simulink model "MCity_cs_withAEBSBlock"  (R2017a)
settings: Solver=ode5  StartTime=0.0  StopTime=3.95  FixedStep=1/200  RelTol=1e-3
PreLoadFcn:
  | check_NUTS_defined;
  | 
  | assignin('base',['model_closed_' bdroot],false);
InitFcn:
  | PreScanExperimentInitFcn(bdroot)
StopFcn:
  | PreScanExperimentStopFcn(bdroot)
model workspace (MAT data in the model file):
  mbox_table : struct (value not decoded)
  model_closed = 0
  sim_status = 0
values from neighbouring files (symbols this model uses):
  d_offset = -18.15    [monocityTestLeftTurn.mat]    (also in simulation_leftTurn_PreScan.m = dl/vl*vh - 43 + R)
undefined symbols (not defined in the file or in its folder): DiscIntNeverNeededParam, warningInitialVelocity, x0
libraries: simulink x78, PreScanSimulinkLibrary x14, simulink_extras x10, PreScanUsefulBlocks x4
(part 1 of 12)
CloseFcn:
  | evalin('base',['clear model_closed_' bdroot]);
settings Model: Creator=PRESCAN  LastModifiedBy=zhaoding
settings DataIOCC: LimitDataPoints=on  SaveFormat=Array
settings OptimizationCC: ExpressionDepthLimit=2147483647  InitFltsAndDblsToZero=on  LifeSpan=inf
settings DebuggingCC: SaveWithParameterizedLinksMsg=none  UnderspecifiedInitializationDetection=Classic  MergeDetectMultiDrivingBlocksExec=none  SignalResolutionControl=TryResolveAllWithWarning  MultiTaskDSMMsg=warning  MultiTaskCondExecSysMsg=none  FcnCallInpInsideContextMsg=warning  StateNameClashWarn=warning  SFUnexpectedBacktrackingDiag=warning  SFNoUnconditionalDefaultTransitionDiag=warning  SFExecutionAtInitializationDiag=none
settings HardwareCC: ProdBitPerPointer=32  ProdBitPerSizeT=32  ProdBitPerPtrDiffT=32  ProdLargestAtomicFloat=None  ProdIntDivRoundTo=Undefined  ProdEndianess=Unspecified  ProdWordSize=32  ProdHWDeviceType=32-bit Generic
settings ModelReferenceCC: PropagateSignalLabelsOutOfModel=off
settings GRTTargetCC: TargetFcnLib=ansi_tfl_tmw.mat  TargetLangStandard=C89/C90 (ANSI)  GeneratePreprocessorConditionals=Disable all  CombineOutputUpdateFcns=off  GRTInterface=on
settings ConfigComp: CovMetricSettings=dw  CovHtmlReporting=on  CovSaveCumulativeToWorkspaceVar=on  CovSaveSingleToWorkspaceVar=on  CovExternalEMLEnable=off

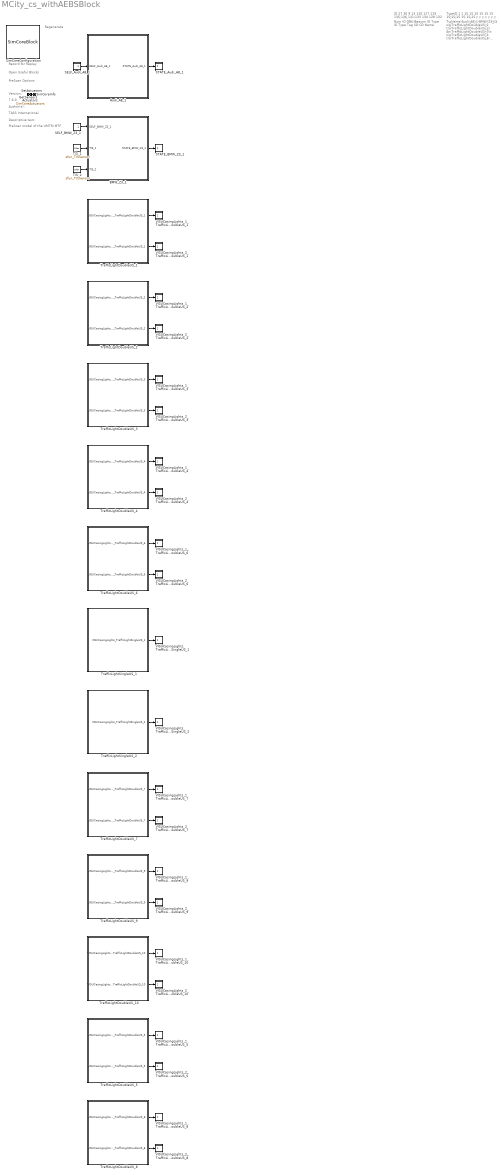
== system MCity_cs_withAEBSBlock ==
  note: Regenerate
  note: Record for Replay
  note: Open Useful Blocks
  note: PreScan Options
  note: Version:
  note: 7.6.0
  note: Author(s):
  note: TASS International
  note: Descriptive text:
  note: PreScan model of the UMTRI MTF.
  note: OBU-Beacon ID
  note: SD
      |
      | Y
      | Y
      | Y
      | Y
      | Y
      | Y
      | Y
      | Y
      | Y
      | Y
      | Y
      | Y
      | Y
      | Y
  note: CD
      |
      | N
      | N
      | N
      | N
      | N
      | N
      | N
      | N
      | N
      | N
      | N
      | N
      | N
      | N
  note: Num ID OBU-Beacon ID Type ID Type Tag SD CD Name
  note: TypeID
      |
      | 1
      | 1
      | 15
      | 15
      | 15
      | 15
      | 15
      | 15
      | 15
      | 15
      | 15
      | 15
      | 15
      | 15
  note: TypeTag
      |
      | Car
      | Car
      | Anim traffic sign
      | Anim traffic sign
      | Anim traffic sign
      | Anim traffic sign
      | Anim traffic sign
      | Anim traffic sign
      | Anim traffic sign
      | Anim traffic sign
      | Anim traffic sign
      | Anim traffic sign
      | Anim traffic sign
      | Anim traffic sign
  note: ID
      |
      | 27
      | 36
      | 9
      | 13
      | 126
      | 127
      | 129
      | 135
      | 136
      | 131
      | 133
      | 134
      | 128
      | 132
  note: Name
      |
      | Audi_A8_1
      | BMW_Z3_1
      | TrafficLightDoubleUS_1
      | TrafficLightDoubleUS_2
      | TrafficLightDoubleUS_3
      | TrafficLightDoubleUS_4
      | TrafficLightDoubleUS_6
      | TrafficLightSingleUS_1
      | TrafficLightSingleUS_2
      | TrafficLightDoubleUS_7
      | TrafficLightDoubleUS_9
      | TrafficLightDoubleUS_10
      | TrafficLightDoubleUS_5
      | TrafficLightDoubleUS_8
  Actuators : DataStoreMemory  Tag=Actuators  DataStoreName=SimCoreActuators  InitialValue=zeros(1086,1)  ShowAdditionalParam=off
      settings: DeleteFcn=PreScanBlockDeleteFcn;
  Audi_A8_1 : Subsystem  Tag=WorldObjectSubSystem  InitFcn=UniqueId = '11817';
      mask Display: image(imread('Audi_A8.jpg'));color('white');text(0,0,' ID=27\n')
  BMW_Z3_1 : Subsystem  Tag=WorldObjectSubSystem  InitFcn=|
      | UniqueId = '12190';
      | UniqueId = '12335';
      mask Display: image(imread('BMW_Z3.jpg'));color('white');text(0,0,' ID=36\n')
  GetSensors : Subsystem  Tag=GetSensors  Priority=2  mask(PreScan Simulation Core Block){NrOfSensors=16, TimeStep=1/200}
      mask prompts: NrOfSensors "Number of sensor values"; TimeStep "Timestep [s]"
      mask help:
      | Please do not remove this block from the PreScan compilation sheet,
      | as it contains essential configuration parameters for a PreScan simulation.
      settings: DeleteFcn=PreScanBlockDeleteFcn;
  SELF_Audi_A8_1 : Subsystem  Tag=SELF  Priority=3  mask(PreScan Source Block: SELF){PortName=SELF_Audi_A8_1, PortIndex=0, PortWidth=8, TimeStep=1/200}
      mask prompts: PortName "Auto-Assigned: Port Name [-]"; PortIndex "Auto-Assigned: Port Index [-]"; PortWidth "Auto-Assigned: Port Dimensions"; TimeStep "Auto-Assigned: Upload Period [s]"
      mask help:
      | The SELF port shows (state) information of the actor itself. The outputs are position in the experiment's axis system and the GPS coordinates, and the object's absolute velocity and compass heading.
      |
      | For more information, please click Help.
      settings: DeleteFcn=PreScanBlockDeleteFcn;
      mask Help: eval('openHelp(462)')
      mask Display: image(imread('GPS.png'))
  SELF_BMW_Z3_1 : Subsystem  Tag=SELF  Priority=3  mask(PreScan Source Block: SELF){PortName=SELF_BMW_Z3_1, PortIndex=8, PortWidth=8, TimeStep=1/200}
      mask prompts: PortName "Auto-Assigned: Port Name [-]"; PortIndex "Auto-Assigned: Port Index [-]"; PortWidth "Auto-Assigned: Port Dimensions"; TimeStep "Auto-Assigned: Upload Period [s]"
      mask help:
      | The SELF port shows (state) information of the actor itself. The outputs are position in the experiment's axis system and the GPS coordinates, and the object's absolute velocity and compass heading.
      |
      | For more information, please click Help.
      settings: DeleteFcn=PreScanBlockDeleteFcn;
      mask Help: eval('openHelp(462)')
      mask Display: image(imread('GPS.png'))
  STATE_Audi_A8_1 : Subsystem  Tag=State  Priority=0  mask(PreScan Sink Block: State){x0=-87.178748857646355, y0=373.9608626085182, z0=0.55, Roll0=0, Pitch0=0, Yaw0=92.476977617278507, TimeStep=1/200}
      mask prompts: x0 "Ini x-position VEHICLE wrt GLOBAL axis system [m]"; y0 "Ini y-position VEHICLE wrt GLOBAL axis system [m]"; z0 "Ini z-position VEHICLE wrt GLOBAL axis system [m]"; Roll0 "Ini roll-angle BODY wrt VEHICLE axis system [deg]"; Pitch0 "Ini pitch-angle BODY wrt VEHICLE axis system [deg]"; Yaw0 "Ini yaw-angle VEHICLE wrt GLOBAL axis system [deg]"; TimeStep "Time Step [s]"
      mask help:
      | The Actor State contains a vector signal of size (9x1), containing the following signals:
      |
      | -  Position                  (x,y,z)                                     [m]
      | -  Velocity                  (vx,vy,vz)                               [m/s]
      | -  Angles                    (Roll, Pitch, Yaw)                   [rad]
      |
      | The Actor state is defined in the global axis system.
      | The state is superponed on the Initial position defined in the GUI.
      |
      | For more information, please click Help.
      settings: DeleteFcn=PreScanBlockDeleteFcn;
      mask Help: eval('openHelp(222)')
      mask Display: image(imread('State.png'))
  STATE_BMW_Z3_1 : Subsystem  Tag=State  Priority=0  mask(PreScan Sink Block: State){x0=-92.980654036561049, y0=432.99562062308286, z0=0.4784, Roll0=0, Pitch0=0, Yaw0=271.20288231302447, TimeStep=1/200}
      mask prompts: x0 "Ini x-position VEHICLE wrt GLOBAL axis system [m]"; y0 "Ini y-position VEHICLE wrt GLOBAL axis system [m]"; z0 "Ini z-position VEHICLE wrt GLOBAL axis system [m]"; Roll0 "Ini roll-angle BODY wrt VEHICLE axis system [deg]"; Pitch0 "Ini pitch-angle BODY wrt VEHICLE axis system [deg]"; Yaw0 "Ini yaw-angle VEHICLE wrt GLOBAL axis system [deg]"; TimeStep "Time Step [s]"
      mask help:
      | The Actor State contains a vector signal of size (9x1), containing the following signals:
      |
      | -  Position                  (x,y,z)                                     [m]
      | -  Velocity                  (vx,vy,vz)                               [m/s]
      | -  Angles                    (Roll, Pitch, Yaw)                   [rad]
      |
      | The Actor state is defined in the global axis system.
      | The state is superponed on the Initial position defined in the GUI.
      |
      | For more information, please click Help.
      settings: DeleteFcn=PreScanBlockDeleteFcn;
      mask Help: eval('openHelp(222)')
      mask Display: image(imread('State.png'))
  SetActuators : Subsystem  Tag=SetActuators  Priority=1  mask(PreScan Simulation Core Block){TimeStep=1/200, NrOfActuators=1086}
      mask prompts: TimeStep "Timestep [s]"; NrOfActuators "Number of actuator values"
      mask help:
      | Please do not remove this block from the PreScan compilation sheet,
      | as it contains essential configuration parameters for a PreScan simulation.
      settings: DeleteFcn=PreScanBlockDeleteFcn;
  SimCoreConfiguration : M-S-Function  Tag=SimCoreConfiguration  Description=6A63ADE35867DA85095F0771801E5CBC5CA8CDFACC45876E9CB8251708310E18  FunctionName=SimCoreBlock  Parameters=ExperimentXML PortsXML SimulationCore HostName CheckStart EnableLog RfR EnableGPUAccel ShowComputationTime  mask(PreScan Simulation Core Configurator){SimulationCore=NUTS, HostName=0, CheckStart=0, prescanversion='7.6.0', EnableLog=off, RfR=0, EnableGPUAccel=off, ShowComputationTime=off}
      mask prompts: SimulationCore "Simulation Core"; HostName "Simulation Host"; CheckStart "Show START Dialog"; prescanversion "PreScan Version"; EnableLog "Create TA Log"; RfR "Record for Replay"; EnableGPUAccel "Enable GPU Acceleration"; ShowComputationTime "Show ComputationTime Scope"
      mask help:
      | Please do not remove this block from the PreScan compilation sheet,
      | as it contains essential configuration parameter for a PreScan simulation.
      mask init:
      | model = bdroot;
      | ExperimentXML = [model(1:end-3) '.pex'];
      | PortsXML = [model '_ports.pcd'];
      settings: DeleteFcn=PreScanBlockDeleteFcn;  ModelCloseFcn=assignin('base',['model_closed_' bdroot],true);
      mask Help: eval('openHelp(812)')
      mask Display: image(imread('prescanlogo.ico'))
  SimCoreInfo : Subsystem  Tag=SimCoreInfo
  TIS_1 : S-Function  Priority=3  LoadFcn=load('PrescanScannerSensorData.mat');load('PrescanScannerSensorMessage.mat')  FunctionName=sfun_TISSensor  Parameters=timestepMask maxInputMessages maxOutputMessages sensorID detectableObjects  SFunctionDeploymentMode=off  EnableBusSupport=off  mask{timestepMask=1/4, maxInputMessages=0, maxOutputMessages=1, sensorID=13179, detectableObjects=1}
      mask prompts: timestepMask "MATLAB timestep:"; maxInputMessages "Max input messages:"; maxOutputMessages "Max output messages:"; sensorID "Sensor ID:"; detectableObjects "Max detectable objects:"
      mask help: TIS Sensor I/O
      mask Display: image(imread('TIS.png'))
  TIS_2 : S-Function  Priority=3  LoadFcn=load('PrescanScannerSensorData.mat');load('PrescanScannerSensorMessage.mat')  FunctionName=sfun_TISSensor  Parameters=timestepMask maxInputMessages maxOutputMessages sensorID detectableObjects  SFunctionDeploymentMode=off  EnableBusSupport=off  mask{timestepMask=1/4, maxInputMessages=0, maxOutputMessages=1, sensorID=13180, detectableObjects=1}
      mask prompts: timestepMask "MATLAB timestep:"; maxInputMessages "Max input messages:"; maxOutputMessages "Max output messages:"; sensorID "Sensor ID:"; detectableObjects "Max detectable objects:"
      mask help: TIS Sensor I/O
      mask Display: image(imread('TIS.png'))
  TrafficLightDoubleUS_1 : Subsystem  Tag=WorldObjectSubSystem  InitFcn=UniqueId = '5551';
      mask Display: image(imread('TrafficLightDoubleUS.jpg'));color('white');text(0,0,' ID=9\n')
  TrafficLightDoubleUS_10 : Subsystem  Tag=WorldObjectSubSystem  InitFcn=UniqueId = '6200';
      mask Display: image(imread('TrafficLightDoubleUS.jpg'));color('white');text(0,0,' ID=134\n')
  TrafficLightDoubleUS_2 : Subsystem  Tag=WorldObjectSubSystem  InitFcn=UniqueId = '5552';
      mask Display: image(imread('TrafficLightDoubleUS.jpg'));color('white');text(0,0,' ID=13\n')
  TrafficLightDoubleUS_3 : Subsystem  Tag=WorldObjectSubSystem  InitFcn=UniqueId = '6076';
      mask Display: image(imread('TrafficLightDoubleUS.jpg'));color('white');text(0,0,' ID=126\n')
  TrafficLightDoubleUS_4 : Subsystem  Tag=WorldObjectSubSystem  InitFcn=UniqueId = '6077';
      mask Display: image(imread('TrafficLightDoubleUS.jpg'));color('white');text(0,0,' ID=127\n')
  TrafficLightDoubleUS_5 : Subsystem  Tag=WorldObjectSubSystem  InitFcn=UniqueId = '6078';
      mask Display: image(imread('TrafficLightDoubleUS.jpg'));color('white');text(0,0,' ID=128\n')
  TrafficLightDoubleUS_6 : Subsystem  Tag=WorldObjectSubSystem  InitFcn=UniqueId = '6079';
      mask Display: image(imread('TrafficLightDoubleUS.jpg'));color('white');text(0,0,' ID=129\n')
  TrafficLightDoubleUS_7 : Subsystem  Tag=WorldObjectSubSystem  InitFcn=UniqueId = '6197';
      mask Display: image(imread('TrafficLightDoubleUS.jpg'));color('white');text(0,0,' ID=131\n')
  TrafficLightDoubleUS_8 : Subsystem  Tag=WorldObjectSubSystem  InitFcn=UniqueId = '6198';
      mask Display: image(imread('TrafficLightDoubleUS.jpg'));color('white');text(0,0,' ID=132\n')
  TrafficLightDoubleUS_9 : Subsystem  Tag=WorldObjectSubSystem  InitFcn=UniqueId = '6199';
      mask Display: image(imread('TrafficLightDoubleUS.jpg'));color('white');text(0,0,' ID=133\n')
  TrafficLightSingleUS_1 : Subsystem  Tag=WorldObjectSubSystem  InitFcn=UniqueId = '6081';
      mask Display: image(imread('TrafficLightSingleUS.jpg'));color('white');text(0,0,' ID=135\n')
  TrafficLightSingleUS_2 : Subsystem  Tag=WorldObjectSubSystem  InitFcn=UniqueId = '6082';
      mask Display: image(imread('TrafficLightSingleUS.jpg'));color('white');text(0,0,' ID=136\n')
  VISUCasingLights_1_TrafficLightDoubleUS_1 : Subsystem  Tag=VisuCasingLights  Priority=0  mask(PreScan Sink Block: VisuLights){}
      mask help:
      | The VisuLights block provides a way to animate the indicator and braking lights of a vehicle.
      |
      | For more information, please click Help.
      settings: DeleteFcn=PreScanBlockDeleteFcn;
      mask Help: eval('openHelp(223)')
      mask Display: image(imread('TrafficLightCasing.png'))
  VISUCasingLights_1_TrafficLightDoubleUS_10 : Subsystem  Tag=VisuCasingLights  Priority=0  mask(PreScan Sink Block: VisuLights){}
      mask help:
      | The VisuLights block provides a way to animate the indicator and braking lights of a vehicle.
      |
      | For more information, please click Help.
      settings: DeleteFcn=PreScanBlockDeleteFcn;
      mask Help: eval('openHelp(223)')
      mask Display: image(imread('TrafficLightCasing.png'))
  VISUCasingLights_1_TrafficLightDoubleUS_2 : Subsystem  Tag=VisuCasingLights  Priority=0  mask(PreScan Sink Block: VisuLights){}
      mask help:
      | The VisuLights block provides a way to animate the indicator and braking lights of a vehicle.
      |
      | For more information, please click Help.
      settings: DeleteFcn=PreScanBlockDeleteFcn;
      mask Help: eval('openHelp(223)')
      mask Display: image(imread('TrafficLightCasing.png'))
  VISUCasingLights_1_TrafficLightDoubleUS_3 : Subsystem  Tag=VisuCasingLights  Priority=0  mask(PreScan Sink Block: VisuLights){}
      mask help:
      | The VisuLights block provides a way to animate the indicator and braking lights of a vehicle.
      |
      | For more information, please click Help.
      settings: DeleteFcn=PreScanBlockDeleteFcn;
      mask Help: eval('openHelp(223)')
      mask Display: image(imread('TrafficLightCasing.png'))
  VISUCasingLights_1_TrafficLightDoubleUS_4 : Subsystem  Tag=VisuCasingLights  Priority=0  mask(PreScan Sink Block: VisuLights){}
      mask help:
      | The VisuLights block provides a way to animate the indicator and braking lights of a vehicle.
      |
      | For more information, please click Help.
      settings: DeleteFcn=PreScanBlockDeleteFcn;
      mask Help: eval('openHelp(223)')
      mask Display: image(imread('TrafficLightCasing.png'))
  VISUCasingLights_1_TrafficLightDoubleUS_5 : Subsystem  Tag=VisuCasingLights  Priority=0  mask(PreScan Sink Block: VisuLights){}
      mask help:
      | The VisuLights block provides a way to animate the indicator and braking lights of a vehicle.
      |
      | For more information, please click Help.
      settings: DeleteFcn=PreScanBlockDeleteFcn;
      mask Help: eval('openHelp(223)')
      mask Display: image(imread('TrafficLightCasing.png'))
  VISUCasingLights_1_TrafficLightDoubleUS_6 : Subsystem  Tag=VisuCasingLights  Priority=0  mask(PreScan Sink Block: VisuLights){}
      mask help:
      | The VisuLights block provides a way to animate the indicator and braking lights of a vehicle.
      |
      | For more information, please click Help.
      settings: DeleteFcn=PreScanBlockDeleteFcn;
      mask Help: eval('openHelp(223)')
      mask Display: image(imread('TrafficLightCasing.png'))
  VISUCasingLights_1_TrafficLightDoubleUS_7 : Subsystem  Tag=VisuCasingLights  Priority=0  mask(PreScan Sink Block: VisuLights){}
      mask help:
      | The VisuLights block provides a way to animate the indicator and braking lights of a vehicle.
      |
      | For more information, please click Help.
      settings: DeleteFcn=PreScanBlockDeleteFcn;
      mask Help: eval('openHelp(223)')
      mask Display: image(imread('TrafficLightCasing.png'))
  VISUCasingLights_1_TrafficLightDoubleUS_8 : Subsystem  Tag=VisuCasingLights  Priority=0  mask(PreScan Sink Block: VisuLights){}
      mask help:
      | The VisuLights block provides a way to animate the indicator and braking lights of a vehicle.
      |
      | For more information, please click Help.
      settings: DeleteFcn=PreScanBlockDeleteFcn;
      mask Help: eval('openHelp(223)')
      mask Display: image(imread('TrafficLightCasing.png'))
  VISUCasingLights_1_TrafficLightDoubleUS_9 : Subsystem  Tag=VisuCasingLights  Priority=0  mask(PreScan Sink Block: VisuLights){}
      mask help:
      | The VisuLights block provides a way to animate the indicator and braking lights of a vehicle.
      |
      | For more information, please click Help.
      settings: DeleteFcn=PreScanBlockDeleteFcn;
      mask Help: eval('openHelp(223)')
      mask Display: image(imread('TrafficLightCasing.png'))
  VISUCasingLights_2_TrafficLightDoubleUS_1 : Subsystem  Tag=VisuCasingLights  Priority=0  mask(PreScan Sink Block: VisuLights){}
      mask help:
      | The VisuLights block provides a way to animate the indicator and braking lights of a vehicle.
      |
      | For more information, please click Help.
      settings: DeleteFcn=PreScanBlockDeleteFcn;
      mask Help: eval('openHelp(223)')
      mask Display: image(imread('TrafficLightCasing.png'))
  VISUCasingLights_2_TrafficLightDoubleUS_10 : Subsystem  Tag=VisuCasingLights  Priority=0  mask(PreScan Sink Block: VisuLights){}
      mask help:
      | The VisuLights block provides a way to animate the indicator and braking lights of a vehicle.
      |
      | For more information, please click Help.
      settings: DeleteFcn=PreScanBlockDeleteFcn;
      mask Help: eval('openHelp(223)')
      mask Display: image(imread('TrafficLightCasing.png'))
  VISUCasingLights_2_TrafficLightDoubleUS_2 : Subsystem  Tag=VisuCasingLights  Priority=0  mask(PreScan Sink Block: VisuLights){}
      mask help:
      | The VisuLights block provides a way to animate the indicator and braking lights of a vehicle.
      |
      | For more information, please click Help.
      settings: DeleteFcn=PreScanBlockDeleteFcn;
      mask Help: eval('openHelp(223)')
      mask Display: image(imread('TrafficLightCasing.png'))
  VISUCasingLights_2_TrafficLightDoubleUS_3 : Subsystem  Tag=VisuCasingLights  Priority=0  mask(PreScan Sink Block: VisuLights){}
      mask help:
      | The VisuLights block provides a way to animate the indicator and braking lights of a vehicle.
      |
      | For more information, please click Help.
      settings: DeleteFcn=PreScanBlockDeleteFcn;
      mask Help: eval('openHelp(223)')
      mask Display: image(imread('TrafficLightCasing.png'))
  VISUCasingLights_2_TrafficLightDoubleUS_4 : Subsystem  Tag=VisuCasingLights  Priority=0  mask(PreScan Sink Block: VisuLights){}
      mask help:
      | The VisuLights block provides a way to animate the indicator and braking lights of a vehicle.
      |
      | For more information, please click Help.
      settings: DeleteFcn=PreScanBlockDeleteFcn;
      mask Help: eval('openHelp(223)')
      mask Display: image(imread('TrafficLightCasing.png'))
  VISUCasingLights_2_TrafficLightDoubleUS_5 : Subsystem  Tag=VisuCasingLights  Priority=0  mask(PreScan Sink Block: VisuLights){}
      mask help:
      | The VisuLights block provides a way to animate the indicator and braking lights of a vehicle.
      |
      | For more information, please click Help.
      settings: DeleteFcn=PreScanBlockDeleteFcn;
      mask Help: eval('openHelp(223)')
      mask Display: image(imread('TrafficLightCasing.png'))
  VISUCasingLights_2_TrafficLightDoubleUS_6 : Subsystem  Tag=VisuCasingLights  Priority=0  mask(PreScan Sink Block: VisuLights){}
      mask help:
      | The VisuLights block provides a way to animate the indicator and braking lights of a vehicle.
      |
      | For more information, please click Help.
      settings: DeleteFcn=PreScanBlockDeleteFcn;
      mask Help: eval('openHelp(223)')
      mask Display: image(imread('TrafficLightCasing.png'))
  VISUCasingLights_2_TrafficLightDoubleUS_7 : Subsystem  Tag=VisuCasingLights  Priority=0  mask(PreScan Sink Block: VisuLights){}
      mask help:
      | The VisuLights block provides a way to animate the indicator and braking lights of a vehicle.
      |
      | For more information, please click Help.
      settings: DeleteFcn=PreScanBlockDeleteFcn;
      mask Help: eval('openHelp(223)')
      mask Display: image(imread('TrafficLightCasing.png'))
  VISUCasingLights_2_TrafficLightDoubleUS_8 : Subsystem  Tag=VisuCasingLights  Priority=0  mask(PreScan Sink Block: VisuLights){}
      mask help:
      | The VisuLights block provides a way to animate the indicator and braking lights of a vehicle.
      |
      | For more information, please click Help.
      settings: DeleteFcn=PreScanBlockDeleteFcn;
      mask Help: eval('openHelp(223)')
      mask Display: image(imread('TrafficLightCasing.png'))
  VISUCasingLights_2_TrafficLightDoubleUS_9 : Subsystem  Tag=VisuCasingLights  Priority=0  mask(PreScan Sink Block: VisuLights){}
      mask help:
      | The VisuLights block provides a way to animate the indicator and braking lights of a vehicle.
      |
      | For more information, please click Help.
      settings: DeleteFcn=PreScanBlockDeleteFcn;
      mask Help: eval('openHelp(223)')
      mask Display: image(imread('TrafficLightCasing.png'))
  VISUCasingLights_TrafficLightSingleUS_1 : Subsystem  Tag=VisuCasingLights  Priority=0  mask(PreScan Sink Block: VisuLights){}
      mask help:
      | The VisuLights block provides a way to animate the indicator and braking lights of a vehicle.
      |
      | For more information, please click Help.
      settings: DeleteFcn=PreScanBlockDeleteFcn;
      mask Help: eval('openHelp(223)')
      mask Display: image(imread('TrafficLightCasing.png'))
  VISUCasingLights_TrafficLightSingleUS_2 : Subsystem  Tag=VisuCasingLights  Priority=0  mask(PreScan Sink Block: VisuLights){}
      mask help:
      | The VisuLights block provides a way to animate the indicator and braking lights of a vehicle.
      |
      | For more information, please click Help.
      settings: DeleteFcn=PreScanBlockDeleteFcn;
      mask Help: eval('openHelp(223)')
      mask Display: image(imread('TrafficLightCasing.png'))
  wires:
  TrafficLightDoubleUS_10/2(VISUCasingLights_2_TrafficLightDoubleUS_10) -> VISUCasingLights_2_TrafficLightDoubleUS_10/1(CasingLights)
  TrafficLightDoubleUS_10/1(VISUCasingLights_1_TrafficLightDoubleUS_10) -> VISUCasingLights_1_TrafficLightDoubleUS_10/1(CasingLights)
  TrafficLightDoubleUS_9/2(VISUCasingLights_2_TrafficLightDoubleUS_9) -> VISUCasingLights_2_TrafficLightDoubleUS_9/1(CasingLights)
  TrafficLightDoubleUS_9/1(VISUCasingLights_1_TrafficLightDoubleUS_9) -> VISUCasingLights_1_TrafficLightDoubleUS_9/1(CasingLights)
  TrafficLightDoubleUS_8/2(VISUCasingLights_2_TrafficLightDoubleUS_8) -> VISUCasingLights_2_TrafficLightDoubleUS_8/1(CasingLights)
  TrafficLightDoubleUS_8/1(VISUCasingLights_1_TrafficLightDoubleUS_8) -> VISUCasingLights_1_TrafficLightDoubleUS_8/1(CasingLights)
  TrafficLightDoubleUS_7/2(VISUCasingLights_2_TrafficLightDoubleUS_7) -> VISUCasingLights_2_TrafficLightDoubleUS_7/1(CasingLights)
  TrafficLightDoubleUS_7/1(VISUCasingLights_1_TrafficLightDoubleUS_7) -> VISUCasingLights_1_TrafficLightDoubleUS_7/1(CasingLights)
  TrafficLightSingleUS_2/1(VISUCasingLights_TrafficLightSingleUS_2) -> VISUCasingLights_TrafficLightSingleUS_2/1(CasingLights)
  TrafficLightSingleUS_1/1(VISUCasingLights_TrafficLightSingleUS_1) -> VISUCasingLights_TrafficLightSingleUS_1/1(CasingLights)
  TrafficLightDoubleUS_6/2(VISUCasingLights_2_TrafficLightDoubleUS_6) -> VISUCasingLights_2_TrafficLightDoubleUS_6/1(CasingLights)
  TrafficLightDoubleUS_6/1(VISUCasingLights_1_TrafficLightDoubleUS_6) -> VISUCasingLights_1_TrafficLightDoubleUS_6/1(CasingLights)
  TrafficLightDoubleUS_5/2(VISUCasingLights_2_TrafficLightDoubleUS_5) -> VISUCasingLights_2_TrafficLightDoubleUS_5/1(CasingLights)
  TrafficLightDoubleUS_5/1(VISUCasingLights_1_TrafficLightDoubleUS_5) -> VISUCasingLights_1_TrafficLightDoubleUS_5/1(CasingLights)
  TrafficLightDoubleUS_4/2(VISUCasingLights_2_TrafficLightDoubleUS_4) -> VISUCasingLights_2_TrafficLightDoubleUS_4/1(CasingLights)
  TrafficLightDoubleUS_4/1(VISUCasingLights_1_TrafficLightDoubleUS_4) -> VISUCasingLights_1_TrafficLightDoubleUS_4/1(CasingLights)
  TrafficLightDoubleUS_3/2(VISUCasingLights_2_TrafficLightDoubleUS_3) -> VISUCasingLights_2_TrafficLightDoubleUS_3/1(CasingLights)
  TrafficLightDoubleUS_3/1(VISUCasingLights_1_TrafficLightDoubleUS_3) -> VISUCasingLights_1_TrafficLightDoubleUS_3/1(CasingLights)
  TrafficLightDoubleUS_2/2(VISUCasingLights_2_TrafficLightDoubleUS_2) -> VISUCasingLights_2_TrafficLightDoubleUS_2/1(CasingLights)
  TrafficLightDoubleUS_2/1(VISUCasingLights_1_TrafficLightDoubleUS_2) -> VISUCasingLights_1_TrafficLightDoubleUS_2/1(CasingLights)
  TrafficLightDoubleUS_1/2(VISUCasingLights_2_TrafficLightDoubleUS_1) -> VISUCasingLights_2_TrafficLightDoubleUS_1/1(CasingLights)
  TrafficLightDoubleUS_1/1(VISUCasingLights_1_TrafficLightDoubleUS_1) -> VISUCasingLights_1_TrafficLightDoubleUS_1/1(CasingLights)
  SetActuators/1(dummy) -> GetSensors/1(dummy)
  Audi_A8_1/1(STATE_Audi_A8_1) -> STATE_Audi_A8_1/1(State)
  SELF_Audi_A8_1/1(U) -> Audi_A8_1/1(SELF_Audi_A8_1)
  BMW_Z3_1/1(STATE_BMW_Z3_1) -> STATE_BMW_Z3_1/1(State)
  SELF_BMW_Z3_1/1(U) -> BMW_Z3_1/1(SELF_BMW_Z3_1)
  TIS_1/1 -> BMW_Z3_1/2(TIS_1)
  TIS_2/1 -> BMW_Z3_1/3(TIS_2)

== system MCity_cs_withAEBSBlock/Audi_A8_1 ==
  SELF_Audi_A8_1 : Inport  Tag=SELFInport
  DesiredVelocity : Constant  Tag=DesiredVelocity  Value=15
  Dynamics_Simple : Subsystem  Tag=Simple_Vehicle_Dynamics  mask(PreScan Block: Simple Dynamics){Migrate=on, TimeStep=1/200, ComputationMode=Continuous_Time}
      mask prompts: Migrate "Migrate. During migration this block will be replaced by a newer one."; TimeStep "Auto assigned: Time Step [s]"; ComputationMode "Computation mode:"
      mask help:
      | The Simple Dynamics Model is selected in the GUI to simulate vehicle dynamics behavior.
      |
      | The Simple Dynamics Model is completely open to the user. The parameters of this model can be set in the Simple Dynamics dialog in the GUI.
      |
      | For more information, please click Help.
      mask init:
      | p = SimpleDyn_pars;
      settings: DeleteFcn=PreScanBlockDeleteFcn;
      mask Help: eval('openHelp(220)')
      mask Display:
      | image(imread('SimpleDyn.png'))
      | port_label('input', 1, '{\delta}_S_t_ _e_e_r [deg]','texmode','on')
      | port_label('input', 2, 'Throttle [%]')
      | port_label('input', 3, 'Brake Pres [bar]')
      | port_label('input', 4, 'V_0 [ms-1]','texmode','on')
      | port_label('input', 5, 'Auto=[0]/Manual=[1]')
      | port_label('input', 6, 'Auto_GearShift')
      | port_label('input', 7, 'Manual_GearShift')
      | port_label('output', 1, 'State')
      | port_label('output', 2, 'Vx [ms-1]')
      | port_label('output', 3, 'Perf Params')
  FromDynamics2PathFollowerBusSelector : BusSelector  OutputSignals=vx_[ms-1],vy_[ms-1]
  Gain : Gain  Gain=2
  Ground_1 : Ground
  Ground_2 : Ground
  Ground_3 : Ground
  InitialVelocity : Constant  Tag=InitialVelocity  Value=15
  Mux : Mux  Inputs=3
  PathFollower_Preview_1 : Subsystem  Tag=PathFollower_Preview  mask(PreScan Block: Path Follower with Preview){Migrate=on, FileName='Trajectory_1.mat', mass=1820, Jzz=3746, length_a=2.94 - 1.77, length_l=2.94, Angle_Max_SteeringWheel=500, PreviewTime=1, DelayTime=0.1, LowSpeedLimit=20, MaxSteeringRate=1200, CSSampleTime=1/200, PFIntegrationFrequency=200}
      mask prompts: Migrate "Migrate. During migration this block will be replaced by a newer one."; FileName "Trajectory Name"; mass "Mass vehicle total [kg]"; Jzz "Inertia vehicle around yaw axis [kg m2]"; length_a "Distance between COG and front axle [m]"; length_l "Length of wheelbase [m]"; Angle_Max_SteeringWheel "Maximum steering wheel angle [deg]"; PreviewTime "Preview time [s]"; DelayTime "Delay time [s]"; LowSpeedLimit "Low-speed limit [km/h]"; MaxSteeringRate "Maximum steering wheel angle rate [deg/s]"; CSSampleTime "Compilation Sheet sample time [s]"; PFIntegrationFrequency "Lateral controller frequency [Hz]"
      mask help:
      | The Path Follower Model is selected in the GUI to simulate driver behavior.
      |
      | For more information, please click Help.
      mask init:
      | load(['trajectories/',eval(FileName)])
      | traject=trajectory';
      | 
      | Traj_x=traject(:,2);
      | Traj_y=traject(:,3);
      | Traj_t=traject(2,1);
      | Traj_v=sqrt(traject(:,8).^2+traject(:,9).^2+traject(:,10).^2);
      | 
      | RefreshCounter = (1/CSSampleTime) / (PFIntegrationFrequency); %Compilation sheet frequency/path follower frequency
      | 
      | blockPath = gcb;
      | 
      | clear traject;
      mask Help: eval('openHelp(233)')
  SELF2PathFollowerMux : Mux  Inputs=3
  SELF_Demux : Subsystem  Tag=DemuxSELF  mask(PreScan Demux Block:){}
      settings: DeleteFcn=PreScanBlockDeleteFcn;
      mask Display:
      | port_label('output',1,'x [m]')
      | port_label('output',2,'y [m]')
      | port_label('output',3,'z [m]','texmode','on')
      | port_label('output',4,'Rotx [deg]','texmode','on')
      | port_label('output',5,'Roty [deg]','texmode','on')
      | port_label('output',6,'Rotz [deg]','texmode','on')
      | port_label('output',7,'GPS lat [deg]','texmode','on')
      | port_label('output',8,'GPS long [deg]','texmode','on')
      | port_label('output',9,'GPS alt [m]','texmode','on')
      | port_label('output',10,'Velocity [m/s]')
      | port_label('output',11,'Heading [deg]')
      | port_label('output',12,'Yaw rate [deg/s]')
  Terminator_{1..11} (11 alike) : Terminator
  Trajectories : Subsystem  Tag=Trajectories  mask(PreScan Source Block: Trajectories){}
      mask help:
      | The Trajectory block contains the trajectories defined in the PreScan Experiment Editor. The output of the trajectory block is the (vehicle) State.
      |
      | For more information, please click Help.
      settings: DeleteFcn=PreScanBlockDeleteFcn;
      mask Help: eval('openHelp(312)')
      mask Display: image(imread('Trajectory.png'));
  pos : Constant  Tag=pos  Value=[-87.178748857646355 373.9608626085182 92.476977617278507]
  steering_ratio : Constant  Tag=steering_ratio  Value=20
  susp_front : Constant  Tag=susp_front  Value=72653
  susp_rear : Constant  Tag=susp_rear  Value=121449
  STATE_Audi_A8_1 : Outport  Tag=StateOutport
  tag scope: LeftTurnVehicle_x_y_velocity=global
  wires:
  PathFollower_Preview_1/1(delta_steerwheel [deg]) -> Gain/1
  SELF_Demux/1(x [m]) -> Mux/1, SELF2PathFollowerMux/1
  SELF_Demux/2(y [m]) -> Mux/2, SELF2PathFollowerMux/2
  SELF_Demux/10(velocity [m/s]) -> Mux/3, PathFollower_Preview_1/6(velocity [m/s])
  Gain/1 -> Dynamics_Simple/1(DeltaSteer_[deg])
  Mux/1 -> [LeftTurnVehicle_x_y_velocity]
  pos/1 -> PathFollower_Preview_1/1(TrajOffset x,y,Y [m,m,deg])
  InitialVelocity/1 -> PathFollower_Preview_1/4(Initial Velocity [m/s])
  DesiredVelocity/1 -> PathFollower_Preview_1/5(Desired Velocity [m/s])
  susp_front/1 -> PathFollower_Preview_1/10(CorneringStiffness_Tyres_Front [N/rad])
  susp_rear/1 -> PathFollower_Preview_1/11(CorneringStiffness_Tyres_Rear [N/rad])
  steering_ratio/1 -> PathFollower_Preview_1/12(steering_ratio[-])
  SELF_Audi_A8_1/1 -> SELF_Demux/1(SELF)
  PathFollower_Preview_1/2(throttle [%]) -> Dynamics_Simple/2(Throttle)
  PathFollower_Preview_1/3(brake pressure [bar]) -> Dynamics_Simple/3(Brake)
  PathFollower_Preview_1/4(v0 [m/s]) -> Dynamics_Simple/4(Initial_Vx_[ms-1])
  PathFollower_Preview_1/5(Auto_GearShift) -> Dynamics_Simple/6(Auto_GearShift)
  SELF_Demux/6(rotz [deg]) -> SELF2PathFollowerMux/3
  SELF2PathFollowerMux/1 -> PathFollower_Preview_1/3(position x,y,Y [m,m,deg])
  Dynamics_Simple/3(Perf_Params) -> [Dynamics2PathFollower]
  [Dynamics2PathFollower] -> FromDynamics2PathFollowerBusSelector/1
  FromDynamics2PathFollowerBusSelector/1 -> PathFollower_Preview_1/7(vx [m/s])  "<vx_[ms-1]>"
  FromDynamics2PathFollowerBusSelector/2 -> PathFollower_Preview_1/8(vy [m/s])  "<vy_[ms-1]>"
  SELF_Demux/12(yaw rate [deg/s]) -> PathFollower_Preview_1/9(Yaw rate [deg/s])
  Dynamics_Simple/1(State) -> STATE_Audi_A8_1/1
  Ground_1/1 -> Dynamics_Simple/5(AutoManual_OnOff)
  Ground_2/1 -> Dynamics_Simple/7(Manual_GearShift)
  Dynamics_Simple/2(Vx [m s-1]) -> Terminator_1/1
  Ground_3/1 -> PathFollower_Preview_1/2(ActorOffset_Left(+) / Right(-) [m])
  PathFollower_Preview_1/6(Actor/Traj_distance [m]) -> Terminator_2/1
  PathFollower_Preview_1/7(Actor/Traj_angle [deg]) -> Terminator_3/1
  SELF_Demux/3(z [m]) -> Terminator_4/1
  SELF_Demux/4(rotx [deg]) -> Terminator_5/1
  SELF_Demux/5(roty [deg]) -> Terminator_6/1
  SELF_Demux/7(GPS lat [deg]) -> Terminator_7/1
  SELF_Demux/8(GPS long [deg]) -> Terminator_8/1
  SELF_Demux/9(GPS alt [m]) -> Terminator_9/1
  SELF_Demux/11(heading [deg]) -> Terminator_10/1
  Trajectories/1(State) -> Terminator_11/1

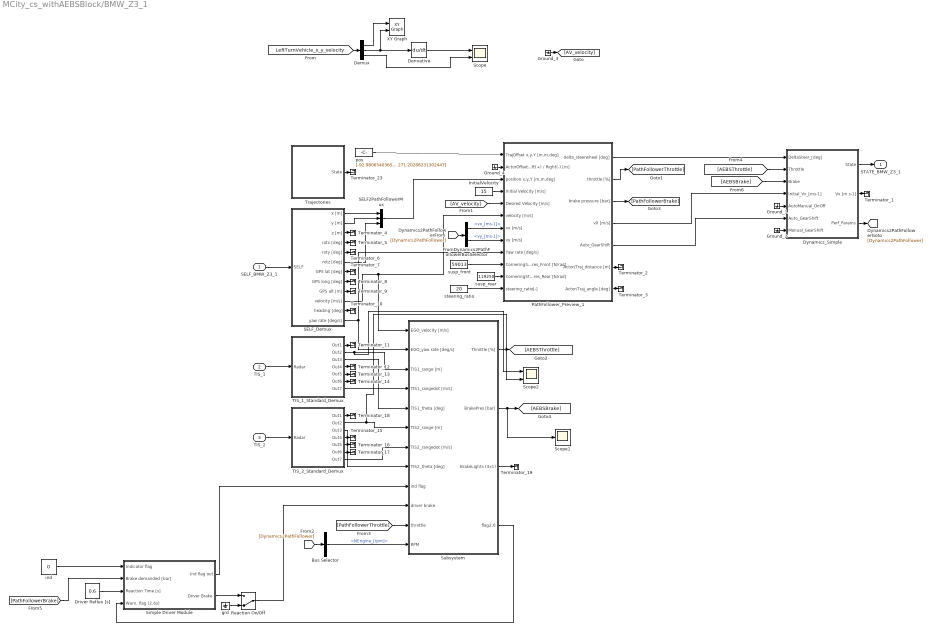
== system MCity_cs_withAEBSBlock/BMW_Z3_1 ==
  SELF_BMW_Z3_1 : Inport  Tag=SELFInport
  TIS_1 : Inport  Tag=RadarInport  Port=2  OutDataTypeStr=Bus: PRESCAN_SCANNERSENSORMESSAGE
  TIS_2 : Inport  Tag=RadarInport  Port=3  OutDataTypeStr=Bus: PRESCAN_SCANNERSENSORMESSAGE
  Bus Selector : BusSelector  OutputSignals=NEngine_[rpm]
  Demux : Demux  Outputs=3
  Derivative : Derivative
  Driver Reflex [s] : Constant  Value=0.6
  Dynamics_Simple : Subsystem  Tag=Simple_Vehicle_Dynamics  mask(PreScan Block: Simple Dynamics){Migrate=on, TimeStep=1/200, ComputationMode=Continuous_Time}
      mask prompts: Migrate "Migrate. During migration this block will be replaced by a newer one."; TimeStep "Auto assigned: Time Step [s]"; ComputationMode "Computation mode:"
      mask help:
      | The Simple Dynamics Model is selected in the GUI to simulate vehicle dynamics behavior.
      |
      | The Simple Dynamics Model is completely open to the user. The parameters of this model can be set in the Simple Dynamics dialog in the GUI.
      |
      | For more information, please click Help.
      mask init:
      | p = SimpleDyn_pars;
      settings: DeleteFcn=PreScanBlockDeleteFcn;
      mask Help: eval('openHelp(220)')
      mask Display:
      | image(imread('SimpleDyn.png'))
      | port_label('input', 1, '{\delta}_S_t_ _e_e_r [deg]','texmode','on')
      | port_label('input', 2, 'Throttle [%]')
      | port_label('input', 3, 'Brake Pres [bar]')
      | port_label('input', 4, 'V_0 [ms-1]','texmode','on')
      | port_label('input', 5, 'Auto=[0]/Manual=[1]')
      | port_label('input', 6, 'Auto_GearShift')
      | port_label('input', 7, 'Manual_GearShift')
      | port_label('output', 1, 'State')
      | port_label('output', 2, 'Vx [ms-1]')
      | port_label('output', 3, 'Perf Params')
  FromDynamics2PathFollowerBusSelector : BusSelector  OutputSignals=vx_[ms-1],vy_[ms-1]
  Ground_{1..4} (4 alike) : Ground
  InitialVelocity : Constant  Tag=InitialVelocity  Value=15
  PathFollower_Preview_1 : Subsystem  Tag=PathFollower_Preview  mask(PreScan Block: Path Follower with Preview){Migrate=on, FileName='Trajectory_2.mat', mass=1435, Jzz=2018, length_a=2.43 - 1.36, length_l=2.43, Angle_Max_SteeringWheel=500, PreviewTime=1, DelayTime=0.1, LowSpeedLimit=20, MaxSteeringRate=1200, CSSampleTime=1/200, PFIntegrationFrequency=200}
      mask prompts: Migrate "Migrate. During migration this block will be replaced by a newer one."; FileName "Trajectory Name"; mass "Mass vehicle total [kg]"; Jzz "Inertia vehicle around yaw axis [kg m2]"; length_a "Distance between COG and front axle [m]"; length_l "Length of wheelbase [m]"; Angle_Max_SteeringWheel "Maximum steering wheel angle [deg]"; PreviewTime "Preview time [s]"; DelayTime "Delay time [s]"; LowSpeedLimit "Low-speed limit [km/h]"; MaxSteeringRate "Maximum steering wheel angle rate [deg/s]"; CSSampleTime "Compilation Sheet sample time [s]"; PFIntegrationFrequency "Lateral controller frequency [Hz]"
      mask help:
      | The Path Follower Model is selected in the GUI to simulate driver behavior.
      |
      | For more information, please click Help.
      mask init: same as MCity_cs_withAEBSBlock/Audi_A8_1/PathFollower_Preview_1
      mask Help: eval('openHelp(233)')
  Reaction On/Off : ManualSwitch  CurrentSetting=0
  SELF2PathFollowerMux : Mux  Inputs=3
  SELF_Demux : Subsystem  Tag=DemuxSELF  mask(PreScan Demux Block:){}
      settings: DeleteFcn=PreScanBlockDeleteFcn;
      mask Display:
      | port_label('output',1,'x [m]')
      | port_label('output',2,'y [m]')
      | port_label('output',3,'z [m]','texmode','on')
      | port_label('output',4,'Rotx [deg]','texmode','on')
      | port_label('output',5,'Roty [deg]','texmode','on')
      | port_label('output',6,'Rotz [deg]','texmode','on')
      | port_label('output',7,'GPS lat [deg]','texmode','on')
      | port_label('output',8,'GPS long [deg]','texmode','on')
      | port_label('output',9,'GPS alt [m]','texmode','on')
      | port_label('output',10,'Velocity [m/s]')
      | port_label('output',11,'Heading [deg]')
      | port_label('output',12,'Yaw rate [deg/s]')
  Scope : Scope  NumInputPorts=2
  Scope1 : Scope
  Scope2 : Scope  NumInputPorts=2
  Simple Driver Module : Subsystem
  Subsystem : Subsystem
  TIS_1_Standard_Demux : Subsystem  TreatAsAtomicUnit=on  mask(PreScan Demux Block: TIS){MAXMESSAGES=1}
      mask prompts: MAXMESSAGES "Number of Objects"
      mask Help: eval('openHelp(441)')
      mask Display:
      | port_label('input',1,'TIS')
      | port_label('output',1,'Beam ID [-]')
      | port_label('output',2,'Range [m]')
      | port_label('output',3,'{\theta} [deg]','texmode','on')
      | port_label('output',4,'{\phi} [deg]','texmode','on')
      | port_label('output',5,'Target ID [-]','texmode','on')
      | port_label('output',6,'TIS Data','texmode','on')
  TIS_2_Standard_Demux : Subsystem  TreatAsAtomicUnit=on  mask(PreScan Demux Block: TIS){MAXMESSAGES=1}
      mask prompts: MAXMESSAGES "Number of Objects"
      mask Help: eval('openHelp(441)')
      mask Display:
      | port_label('input',1,'TIS')
      | port_label('output',1,'Beam ID [-]')
      | port_label('output',2,'Range [m]')
      | port_label('output',3,'{\theta} [deg]','texmode','on')
      | port_label('output',4,'{\phi} [deg]','texmode','on')
      | port_label('output',5,'Target ID [-]','texmode','on')
      | port_label('output',6,'TIS Data','texmode','on')
  Terminator_{1..19,23} (20 alike) : Terminator
  Trajectories : Subsystem  Tag=Trajectories  mask(PreScan Source Block: Trajectories){}
      mask help:
      | The Trajectory block contains the trajectories defined in the PreScan Experiment Editor. The output of the trajectory block is the (vehicle) State.
      |
      | For more information, please click Help.
      settings: DeleteFcn=PreScanBlockDeleteFcn;
      mask Help: eval('openHelp(312)')
      mask Display: image(imread('Trajectory.png'));
  XY Graph : simulink/Sinks/XY Graph  xmin=-142  xmax=-40  ymin=373  ymax=458  st=-1
  grd : Ground
  ind : Constant  Value=0
  pos : Constant  Tag=pos  Value=[-92.980654036561049 432.99562062308286 271.20288231302447]
  steering_ratio : Constant  Tag=steering_ratio  Value=20
  susp_front : Constant  Tag=susp_front  Value=59013
  susp_rear : Constant  Tag=susp_rear  Value=119250
  STATE_BMW_Z3_1 : Outport  Tag=StateOutport
  wires:
  [LeftTurnVehicle_x_y_velocity] -> Demux/1
  Demux/2 -> Derivative/1, XY Graph/2
  Demux/3 -> Scope/2
  Derivative/1 -> Scope/1
  Demux/1 -> XY Graph/1
  [AV_velocity] -> PathFollower_Preview_1/5(Desired Velocity [m/s])
  Subsystem/1(Throttle [%]) -> [AEBSThrottle]
  Subsystem/2(BrakePres [bar]) -> Scope1/1, [AEBSBrake]
  Subsystem/3(BrakeLights (3x1)) -> Terminator_19/1
  pos/1 -> PathFollower_Preview_1/1(TrajOffset x,y,Y [m,m,deg])
  InitialVelocity/1 -> PathFollower_Preview_1/4(Initial Velocity [m/s])
  susp_front/1 -> PathFollower_Preview_1/10(CorneringStiffness_Tyres_Front [N/rad])
  susp_rear/1 -> PathFollower_Preview_1/11(CorneringStiffness_Tyres_Rear [N/rad])
  steering_ratio/1 -> PathFollower_Preview_1/12(steering_ratio[-])
  SELF_BMW_Z3_1/1 -> SELF_Demux/1(SELF)
  TIS_1/1 -> TIS_1_Standard_Demux/1(Radar)
  TIS_2/1 -> TIS_2_Standard_Demux/1(Radar)
  PathFollower_Preview_1/1(delta_steerwheel [deg]) -> Dynamics_Simple/1(DeltaSteer_[deg])
  PathFollower_Preview_1/4(v0 [m/s]) -> Dynamics_Simple/4(Initial_Vx_[ms-1])
  PathFollower_Preview_1/5(Auto_GearShift) -> Dynamics_Simple/6(Auto_GearShift)
  SELF_Demux/1(x [m]) -> SELF2PathFollowerMux/1
  SELF_Demux/2(y [m]) -> SELF2PathFollowerMux/2
  SELF_Demux/6(rotz [deg]) -> SELF2PathFollowerMux/3
  SELF2PathFollowerMux/1 -> PathFollower_Preview_1/3(position x,y,Y [m,m,deg])
  Dynamics_Simple/3(Perf_Params) -> [Dynamics2PathFollower]
  [Dynamics2PathFollower] -> FromDynamics2PathFollowerBusSelector/1
  FromDynamics2PathFollowerBusSelector/1 -> PathFollower_Preview_1/7(vx [m/s])  "<vx_[ms-1]>"
  FromDynamics2PathFollowerBusSelector/2 -> PathFollower_Preview_1/8(vy [m/s])  "<vy_[ms-1]>"
  Dynamics_Simple/1(State) -> STATE_BMW_Z3_1/1
  Ground_1/1 -> Dynamics_Simple/5(AutoManual_OnOff)
  Ground_2/1 -> Dynamics_Simple/7(Manual_GearShift)
  Dynamics_Simple/2(Vx [m s-1]) -> Terminator_1/1
  Ground_3/1 -> [AV_velocity]
  Ground_4/1 -> PathFollower_Preview_1/2(ActorOffset_Left(+) / Right(-) [m])
  PathFollower_Preview_1/6(Actor/Traj_distance [m]) -> Terminator_2/1
  PathFollower_Preview_1/7(Actor/Traj_angle [deg]) -> Terminator_3/1
  SELF_Demux/3(z [m]) -> Terminator_4/1
  SELF_Demux/4(rotx [deg]) -> Terminator_5/1
  SELF_Demux/5(roty [deg]) -> Terminator_6/1
  SELF_Demux/7(GPS lat [deg]) -> Terminator_7/1
  SELF_Demux/8(GPS long [deg]) -> Terminator_8/1
  SELF_Demux/9(GPS alt [m]) -> Terminator_9/1
  SELF_Demux/11(heading [deg]) -> Terminator_10/1
  SELF_Demux/10(velocity [m/s]) -> PathFollower_Preview_1/6(velocity [m/s]), Subsystem/1(EGO_velocity [m/s])
  SELF_Demux/12(yaw rate [deg/s]) -> Subsystem/2(EGO_yaw rate [deg/s]), PathFollower_Preview_1/9(Yaw rate [deg/s])
  TIS_1_Standard_Demux/2(Out2) -> Scope2/1, Subsystem/3(TIS1_range [m])
  TIS_1_Standard_Demux/7(Out7) -> Subsystem/4(TIS1_rangedot [m/s])
  TIS_1_Standard_Demux/3(Out3) -> Subsystem/5(TIS1_theta [deg])
  TIS_2_Standard_Demux/2(Out2) -> Scope2/2, Subsystem/6(TIS2_range [m])
  TIS_2_Standard_Demux/7(Out7) -> Subsystem/7(TIS2_rangedot [m/s])
  TIS_2_Standard_Demux/3(Out3) -> Subsystem/8(TIS2_theta [deg])
  Reaction On/Off/1 -> Subsystem/10(driver brake)
  [PathFollowerThrottle] -> Subsystem/11(throttle)
  Trajectories/1(State) -> Terminator_23/1
  TIS_1_Standard_Demux/1(Out1) -> Terminator_11/1
  TIS_1_Standard_Demux/4(Out4) -> Terminator_12/1
  TIS_1_Standard_Demux/5(Out5) -> Terminator_13/1
  TIS_1_Standard_Demux/6(Out6) -> Terminator_14/1
  TIS_2_Standard_Demux/5(Out5) -> Terminator_16/1
  TIS_2_Standard_Demux/4(Out4) -> Terminator_15/1
  TIS_2_Standard_Demux/6(Out6) -> Terminator_17/1
  TIS_2_Standard_Demux/1(Out1) -> Terminator_18/1
  [Dynamics2PathFollower] -> Bus Selector/1
  Bus Selector/1 -> Subsystem/12(RPM)  "<NEngine_[rpm]>"
  PathFollower_Preview_1/2(throttle [%]) -> [PathFollowerThrottle]
  [AEBSThrottle] -> Dynamics_Simple/2(Throttle)
  grd/1 -> Reaction On/Off/2
  Driver Reflex [s]/1 -> Simple Driver Module/3(Reaction Time [s])
  Simple Driver Module/2(Driver Brake) -> Reaction On/Off/1
  [PathFollowerBrake] -> Simple Driver Module/2(Brake demanded [bar])
  ind/1 -> Simple Driver Module/1(Indicator flag)
  Subsystem/4(flag2.6) -> Simple Driver Module/4(Warn. flag (2.6s))
  Simple Driver Module/1(Ind flag out) -> Subsystem/9(ind flag)
  PathFollower_Preview_1/3(brake pressure [bar]) -> [PathFollowerBrake]
  [AEBSBrake] -> Dynamics_Simple/3(Brake)

== system MCity_cs_withAEBSBlock/GetSensors ==
  dummy : Inport
  GetSensors : M-S-Function  FunctionName=GetSensorsBlock  Parameters=TimeStep NrOfSensors
  tag scope: SimCoreSensors=global
  wires:
  GetSensors/1 -> [SimCoreSensors]
  dummy/1 -> GetSensors/1

== system MCity_cs_withAEBSBlock/SELF_Audi_A8_1 ==
  Selector : Selector  IndexMode=Zero-based  IndexOptions=Starting index (dialog)  Indices=PortIndex  OutputSizes=PortWidth(1)
  U : Outport
  wires:
  Selector/1 -> U/1
  [SimCoreSensors] -> Selector/1

== system MCity_cs_withAEBSBlock/SELF_BMW_Z3_1 ==
  Selector : Selector  IndexMode=Zero-based  IndexOptions=Starting index (dialog)  Indices=PortIndex  OutputSizes=PortWidth(1)
  U : Outport
  wires:
  Selector/1 -> U/1
  [SimCoreSensors] -> Selector/1

== system MCity_cs_withAEBSBlock/STATE_Audi_A8_1 ==
  State : Inport  SampleTime=TimeStep
  Acceleration : Subsystem  mask(ToSensorWorld){PortName=Acceleration_Audi_A8_1, PortIndex=6, PortWidth=3, TimeStep=1/200}
      mask prompts: PortName "Port Name [-]"; PortIndex "Index [-]"; PortWidth "Port Dimensions [-]"; TimeStep "Upload Period [s]"
      mask help: Sends signal(s) from Simulink to the Sensor World
      mask Help:
      | Sends signal(s) from Simulink to the Sensor World.
      | 
      | - Port Name [-]: specifies the name of the output terminal of the Simulink block.
      | - Index [-]: specifies the start position in the output vector sent to the Sensor World
      | - Port dimensions [-]: specifies the width (number of scalars) of the output port
      | - Upload period [s]: specifies the upload period (in seconds) of the port.
      mask Display: port_label('input', 1, PortName)
  Demux : Demux  Outputs=5
  Position : Subsystem  mask(ToSensorWorld){PortName=Position_Audi_A8_1, PortIndex=0, PortWidth=3, TimeStep=1/200}
      mask prompts: PortName "Port Name [-]"; PortIndex "Index [-]"; PortWidth "Port Dimensions [-]"; TimeStep "Upload Period [s]"
      mask help: Sends signal(s) from Simulink to the Sensor World
      mask Help:
      | Sends signal(s) from Simulink to the Sensor World.
      | 
      | - Port Name [-]: specifies the name of the output terminal of the Simulink block.
      | - Index [-]: specifies the start position in the output vector sent to the Sensor World
      | - Port dimensions [-]: specifies the width (number of scalars) of the output port
      | - Upload period [s]: specifies the upload period (in seconds) of the port.
      mask Display: port_label('input', 1, PortName)
  RPY : Subsystem  mask(ToSensorWorld){PortName=RPY_Audi_A8_1, PortIndex=9, PortWidth=3, TimeStep=1/200}
      mask prompts: PortName "Port Name [-]"; PortIndex "Index [-]"; PortWidth "Port Dimensions [-]"; TimeStep "Upload Period [s]"
      mask help: Sends signal(s) from Simulink to the Sensor World
      mask Help:
      | Sends signal(s) from Simulink to the Sensor World.
      | 
      | - Port Name [-]: specifies the name of the output terminal of the Simulink block.
      | - Index [-]: specifies the start position in the output vector sent to the Sensor World
      | - Port dimensions [-]: specifies the width (number of scalars) of the output port
      | - Upload period [s]: specifies the upload period (in seconds) of the port.
      mask Display: port_label('input', 1, PortName)
  Velocity : Subsystem  mask(ToSensorWorld){PortName=Velocity_Audi_A8_1, PortIndex=3, PortWidth=3, TimeStep=1/200}
      mask prompts: PortName "Port Name [-]"; PortIndex "Index [-]"; PortWidth "Port Dimensions [-]"; TimeStep "Upload Period [s]"
      mask help: Sends signal(s) from Simulink to the Sensor World
      mask Help:
      | Sends signal(s) from Simulink to the Sensor World.
      | 
      | - Port Name [-]: specifies the name of the output terminal of the Simulink block.
      | - Index [-]: specifies the start position in the output vector sent to the Sensor World
      | - Port dimensions [-]: specifies the width (number of scalars) of the output port
      | - Upload period [s]: specifies the upload period (in seconds) of the port.
      mask Display: port_label('input', 1, PortName)
  iniBODYAngles wrtVEH [rad] : Constant  Value=[Roll0 Pitch0 0]  SampleTime=TimeStep
  iniVEHAngles wrtGLOB [rad] : Constant  Value=[0 0 Yaw0]  SampleTime=TimeStep
  iniVEHposition wrtGLOB [m] : Constant  Value=[x0 y0 z0]  SampleTime=TimeStep
  state2FullState : PreScanSimulinkLibrary/state2FullState  SystemSampleTime=-1
  velRPY : Subsystem  mask(ToSensorWorld){PortName=velRPY_Audi_A8_1, PortIndex=12, PortWidth=3, TimeStep=1/200}
      mask prompts: PortName "Port Name [-]"; PortIndex "Index [-]"; PortWidth "Port Dimensions [-]"; TimeStep "Upload Period [s]"
      mask help: Sends signal(s) from Simulink to the Sensor World
      mask Help:
      | Sends signal(s) from Simulink to the Sensor World.
      | 
      | - Port Name [-]: specifies the name of the output terminal of the Simulink block.
      | - Index [-]: specifies the start position in the output vector sent to the Sensor World
      | - Port dimensions [-]: specifies the width (number of scalars) of the output port
      | - Upload period [s]: specifies the upload period (in seconds) of the port.
      mask Display: port_label('input', 1, PortName)
  wires:
  Demux/5 -> velRPY/1(Y)
  Demux/4 -> RPY/1(Y)
  Demux/3 -> Acceleration/1(Y)
  Demux/2 -> Velocity/1(Y)
  Demux/1 -> Position/1(Y)
  State/1 -> state2FullState/1
  state2FullState/1 -> Demux/1
  iniVEHposition wrtGLOB [m]/1 -> state2FullState/2
  iniBODYAngles wrtVEH [rad]/1 -> state2FullState/3
  iniVEHAngles wrtGLOB [rad]/1 -> state2FullState/4
